simulink model "scheme_pos_control_yawcontrol"  (R2025a)
settings: Solver=ode3  StartTime=0.0  StopTime=40  FixedStep=dt  RelTol=1e-3
values from neighbouring files (symbols this model uses):
  dt = 0.0005    [Planning_Sim.m]
  goal_pos = waypoints(end, :)'    [Planning_Sim.m]
  initial_positions_rad = rawJointPositions(1, :)'    [manipulator_sim.m]
  manipulator_position_data = positions_final    [manipulator_sim.m]
  manipulator_time_vector = time_final    [manipulator_sim.m]
  map_scale = 0.5    [Planning_Sim.m]
  op_space_pose_trajectory = zeros(4, 4, num_points)    [Planning_Sim.m]
  waypoints = pathObj.States(:, 1:2)    [Planning_Sim.m]
  x0 = zeros(14, 1)    [Planning_Sim.m]
undefined symbols (not defined in the file or in its folder): control_params, p, X, Y, Z
libraries: sm_lib x179, nesl_utility x28, fl_lib x3
(part 1 of 5)
settings Model: SimulationMode=accelerator  Creator=robyr  LastModifiedBy=robyr
settings SolverCC: MinimalZcImpactIntegration=on
settings DebuggingCC: ReadBeforeWriteMsg=DisableAll  WriteAfterWriteMsg=DisableAll  WriteAfterReadMsg=DisableAll  MultiTaskDSMMsg=none
settings ModelReferenceCC: UpdateModelReferenceTargets=IfOutOfDate
settings SFSimCC: SFSimEcho=off
settings ExplorerConfigSet: InternalSimMechanicsExplorerSettings="<ExplorerConfiguration><canonicalview>default</canonicalview><TilePanel><TileInfo><Tiles Columns=\"1\" Count=\"1\" Height=\"983\" Rows=\"1\" Width=\"1140\"><Row Weight=\"1\"/><Column Weight=\"1\"/><Tile Height=\"1\" Width=\"1\" X=\"0\" Y=\"0\"/></Tiles></TileInfo><SceneInfo><SceneViewer><IsThisViewStd><IsStandardView>off</IsStandardView><StandardViewName>Front</StandardViewName></IsThisViewStd><BGColor><R>1</R><G>1</G><B>1</B><A>1</A></BGColor><Camera><DoPerspective>off</DoPerspective><Position><X>16.516580000000001</X><Y>-15.49729</Y><Z>6.32498</Z></Position><Center><X>0.84182000000000001</X><Y>-0.041480000000000003</Y><Z>0.82340999999999998</Z></Center><Up><X>0.26359755665786838</X><Y>0.54953240075907739</Y><Z>0.79279913511555156</Z></Up><XLim>1.6166905375218092</XLim><YLim>1.6166905375218092</YLim><ViewLimDist>0.01</ViewLimDist></Camera></SceneViewer></SceneInfo></TilePanel><MechEditorPanel><GfxPanelCameraMap/><Cameras/><VideoCreator><IncludeTiles>All</IncludeTiles><IncludeTime>on</IncludeTime><IncludeWorldFrame>off</IncludeWorldFrame><PlaybackSpeedRatio>1</PlaybackSpeedRatio><FrameRate>30</FrameRate><FrameSize>auto</FrameSize><VideoFormat>UncompressedAVI</VideoFormat></VideoCreator></MechEditorPanel><PlaybackSettings><PlaybackSpeedFactor>4</PlaybackSpeedFactor></PlaybackSettings></ExplorerConfiguration>"

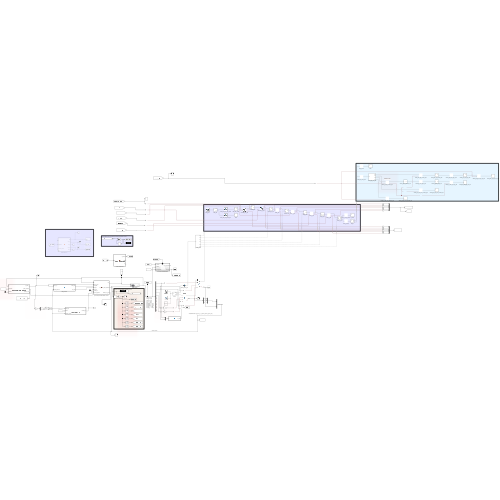
[thumbnail: Simulink's stored preview of the top-level diagram]
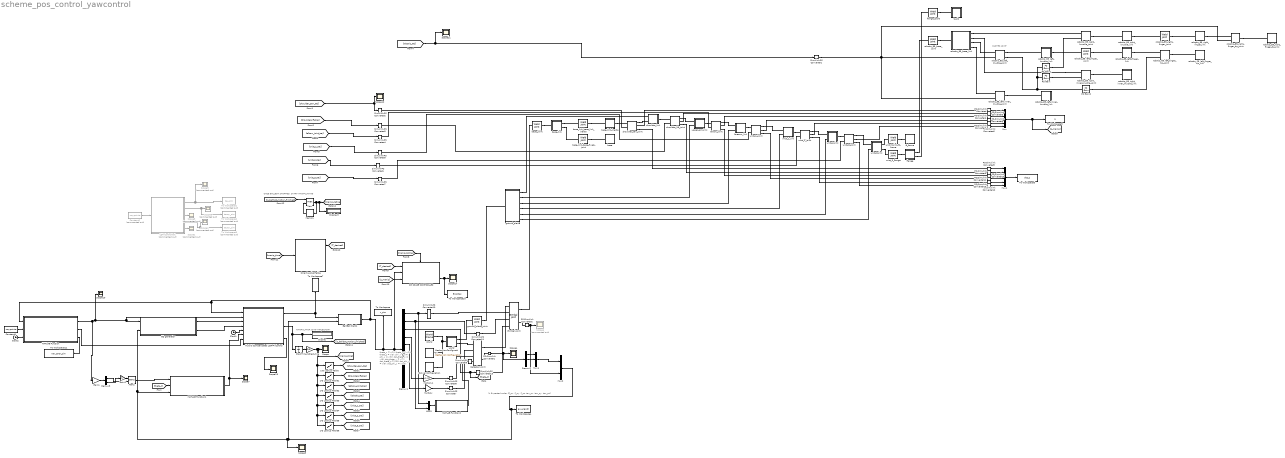
== system scheme_pos_control_yawcontrol ==
  note: MANIPULATOR JOINT TRAJECTORY
  note: % Expected order: [F_px, F_py, F_pz, tau_px, tau_py, tau_pz]
  note: theta_x = x(1);
      | theta_y = x(2);
      | theta_z = x(3);
      | phi_x = x(4);
      | phi_y = x(5);
      | dot_theta_x = x(6);
      | dot_theta_y = x(7);
      | dot_theta_z = x(8);
      | dot_phi_x = x(9);
      | dot_phi_y = x(10);
  note: MASTER JOINT
  note: ONCE BALLBOT STOPPED, START MANIPULATING
  1-D Lookup Table : Lookup_n-D  NumberOfTableDimensions=1  BreakpointsForDimension1=manipulator_time_vector  Table=manipulator_position_data(:,1)  InternalRulePriority=Speed  RndMeth=Simplest
  1-D Lookup Table1 : Lookup_n-D  NumberOfTableDimensions=1  BreakpointsForDimension1=manipulator_time_vector  Table=manipulator_position_data(:,2)  InternalRulePriority=Speed  RndMeth=Simplest
  1-D Lookup Table2 : Lookup_n-D  NumberOfTableDimensions=1  BreakpointsForDimension1=manipulator_time_vector  Table=manipulator_position_data(:,3)  InternalRulePriority=Speed  RndMeth=Simplest
  1-D Lookup Table3 : Lookup_n-D  NumberOfTableDimensions=1  BreakpointsForDimension1=manipulator_time_vector  Table=manipulator_position_data(:,4)  InternalRulePriority=Speed  RndMeth=Simplest
  1-D Lookup Table4 : Lookup_n-D  NumberOfTableDimensions=1  BreakpointsForDimension1=manipulator_time_vector  Table=manipulator_position_data(:,5)  InternalRulePriority=Speed  RndMeth=Simplest
  1-D Lookup Table5 : Lookup_n-D  NumberOfTableDimensions=1  BreakpointsForDimension1=manipulator_time_vector  Table=manipulator_position_data(:,6)  InternalRulePriority=Speed  RndMeth=Simplest
  1-D Lookup Table6 : Lookup_n-D  NumberOfTableDimensions=1  BreakpointsForDimension1=manipulator_time_vector  Table=manipulator_position_data(:,7)  InternalRulePriority=Speed  RndMeth=Simplest
  Atan2 : Trigonometry  Operator=atan2
  BallBot Plant1 : Subsystem
  Cartesian Joint : sm_lib/Joints/Cartesian Joint  JointMode=Normal  CompositeWrenchDir=FollowerOnBase  CompositeWrenchFrame=BaseFrame  SenseConstraintForce=off  SenseConstraintTorque=off  SenseTotalForce=on  SenseTotalTorque=off  PxPositionTargetSpecify=on  PxPositionTargetPriority=High  PxPositionTargetValue=0  PxPositionTargetValueUnits=m  PxVelocityTargetSpecify=on  PxVelocityTargetPriority=High  PxVelocityTargetValue=0  PxVelocityTargetValueUnits=m/s  PxEquilibriumPosition=0  PxEquilibriumPositionUnits=m  PxSpringStiffness=0  PxSpringStiffnessUnits=N/m  PxDampingCoefficient=0  PxDampingCoefficientUnits=N/(m/s)  PxLowerLimitSpecify=off  PxLowerLimitBound=-1  PxLowerLimitBoundUnits=m  PxLowerLimitStiffness=1e6  PxLowerLimitStiffnessUnits=N/m  PxLowerLimitDamping=1e3  PxLowerLimitDampingUnits=N/(m/s)  PxLowerLimitTransitionRegionWidth=1e-4  PxLowerLimitTransitionRegionWidthUnits=m  PxUpperLimitSpecify=off  PxUpperLimitBound=1  PxUpperLimitBoundUnits=m  PxUpperLimitStiffness=1e6  PxUpperLimitStiffnessUnits=N/m  PxUpperLimitDamping=1e3  PxUpperLimitDampingUnits=N/(m/s)  PxUpperLimitTransitionRegionWidth=1e-4  PxUpperLimitTransitionRegionWidthUnits=m  PxTorqueActuationMode=ComputedTorque  PxMotionActuationMode=InputMotion  PxSensePosition=off  PxSenseVelocity=off  PxSenseAcceleration=off  PxSenseTorqueForce=off  PxSenseLowerLimitTorqueForce=off  PxSenseUpperLimitTorqueForce=off  PyPositionTargetSpecify=on  PyPositionTargetPriority=High  PyPositionTargetValue=0  PyPositionTargetValueUnits=m  PyVelocityTargetSpecify=on  PyVelocityTargetPriority=High  PyVelocityTargetValue=0  PyVelocityTargetValueUnits=m/s  PyEquilibriumPosition=0  PyEquilibriumPositionUnits=m  PySpringStiffness=0  PySpringStiffnessUnits=N/m  PyDampingCoefficient=0  PyDampingCoefficientUnits=N/(m/s)  PyLowerLimitSpecify=off  PyLowerLimitBound=-1  PyLowerLimitBoundUnits=m  PyLowerLimitStiffness=1e6  PyLowerLimitStiffnessUnits=N/m  PyLowerLimitDamping=1e3  PyLowerLimitDampingUnits=N/(m/s)  PyLowerLimitTransitionRegionWidth=1e-4  PyLowerLimitTransitionRegionWidthUnits=m  PyUpperLimitSpecify=off  PyUpperLimitBound=1  PyUpperLimitBoundUnits=m  PyUpperLimitStiffness=1e6  PyUpperLimitStiffnessUnits=N/m  PyUpperLimitDamping=1e3  PyUpperLimitDampingUnits=N/(m/s)  PyUpperLimitTransitionRegionWidth=1e-4  PyUpperLimitTransitionRegionWidthUnits=m  PyTorqueActuationMode=ComputedTorque  PyMotionActuationMode=InputMotion  PySensePosition=off  PySenseVelocity=off  PySenseAcceleration=off  PySenseTorqueForce=off  PySenseLowerLimitTorqueForce=off  PySenseUpperLimitTorqueForce=off  PzPositionTargetSpecify=on  PzPositionTargetPriority=High  PzPositionTargetValue=0  PzPositionTargetValueUnits=m  PzVelocityTargetSpecify=on  PzVelocityTargetPriority=High  PzVelocityTargetValue=0  PzVelocityTargetValueUnits=m/s  PzEquilibriumPosition=0  PzEquilibriumPositionUnits=m  PzSpringStiffness=0  PzSpringStiffnessUnits=N/m  PzDampingCoefficient=0  PzDampingCoefficientUnits=N/(m/s)  PzLowerLimitSpecify=off  PzLowerLimitBound=-1  PzLowerLimitBoundUnits=m  PzLowerLimitStiffness=1e6  PzLowerLimitStiffnessUnits=N/m  PzLowerLimitDamping=1e3  PzLowerLimitDampingUnits=N/(m/s)  PzLowerLimitTransitionRegionWidth=1e-4  PzLowerLimitTransitionRegionWidthUnits=m  PzUpperLimitSpecify=off  PzUpperLimitBound=1  PzUpperLimitBoundUnits=m  PzUpperLimitStiffness=1e6  PzUpperLimitStiffnessUnits=N/m  PzUpperLimitDamping=1e3  PzUpperLimitDampingUnits=N/(m/s)  PzUpperLimitTransitionRegionWidth=1e-4  PzUpperLimitTransitionRegionWidthUnits=m  PzTorqueActuationMode=ComputedTorque  PzMotionActuationMode=InputMotion  PzSensePosition=off  PzSenseVelocity=off  PzSenseAcceleration=off  PzSenseTorqueForce=off  PzSenseLowerLimitTorqueForce=off  PzSenseUpperLimitTorqueForce=off
  Clock : Integrator
  Clock1 : Clock
  Clock2 : Clock
  Constant1 : Constant  Value=waypoints
  Constant6 : Constant  Commented=on  Value=waypoints
  Demux1 : Demux  Outputs=10
  Demux2 : Demux  Outputs=3
  Demux3 : Demux  Outputs=2
  Display : Display
  Display3 : Display
  EQ generator : MATLAB Function  TreatAsAtomicUnit=on
  Gain1 : Gain  Gain=p.r_S
  Gain2 : Gain
  Gimbal Joint : sm_lib/Joints/Gimbal Joint  JointMode=Normal  CompositeWrenchDir=FollowerOnBase  CompositeWrenchFrame=BaseFrame  SenseConstraintForce=off  SenseConstraintTorque=off  SenseTotalForce=off  SenseTotalTorque=on  RxPositionTargetSpecify=on  RxPositionTargetPriority=High  RxPositionTargetValue=0  RxPositionTargetValueUnits=deg  RxVelocityTargetSpecify=on  RxVelocityTargetPriority=High  RxVelocityTargetValue=0  RxVelocityTargetValueUnits=deg/s  RxEquilibriumPosition=0  RxEquilibriumPositionUnits=deg  RxSpringStiffness=0  RxSpringStiffnessUnits=N*m/deg  RxDampingCoefficient=0  RxDampingCoefficientUnits=N*m/(deg/s)  RxLowerLimitSpecify=off  RxLowerLimitBound=-90  RxLowerLimitBoundUnits=deg  RxLowerLimitStiffness=1e4  RxLowerLimitStiffnessUnits=N*m/deg  RxLowerLimitDamping=10  RxLowerLimitDampingUnits=N*m/(deg/s)  RxLowerLimitTransitionRegionWidth=0.1  RxLowerLimitTransitionRegionWidthUnits=deg  RxUpperLimitSpecify=off  RxUpperLimitBound=90  RxUpperLimitBoundUnits=deg  RxUpperLimitStiffness=1e4  RxUpperLimitStiffnessUnits=N*m/deg  RxUpperLimitDamping=10  RxUpperLimitDampingUnits=N*m/(deg/s)  RxUpperLimitTransitionRegionWidth=0.1  RxUpperLimitTransitionRegionWidthUnits=deg  RxTorqueActuationMode=ComputedTorque  RxMotionActuationMode=InputMotion  RxSensePosition=off  RxSenseVelocity=off  RxSenseAcceleration=off  RxSenseTorqueForce=off  RxSenseLowerLimitTorqueForce=off  RxSenseUpperLimitTorqueForce=off  RyPositionTargetSpecify=on  RyPositionTargetPriority=High  RyPositionTargetValue=0  RyPositionTargetValueUnits=deg  RyVelocityTargetSpecify=on  RyVelocityTargetPriority=High  RyVelocityTargetValue=0  RyVelocityTargetValueUnits=deg/s  RyEquilibriumPosition=0  RyEquilibriumPositionUnits=deg  RySpringStiffness=0  RySpringStiffnessUnits=N*m/deg  RyDampingCoefficient=0  RyDampingCoefficientUnits=N*m/(deg/s)  RyLowerLimitSpecify=off  RyLowerLimitBound=-90  RyLowerLimitBoundUnits=deg  RyLowerLimitStiffness=1e4  RyLowerLimitStiffnessUnits=N*m/deg  RyLowerLimitDamping=10  RyLowerLimitDampingUnits=N*m/(deg/s)  RyLowerLimitTransitionRegionWidth=0.1  RyLowerLimitTransitionRegionWidthUnits=deg  RyUpperLimitSpecify=off  RyUpperLimitBound=90  RyUpperLimitBoundUnits=deg  RyUpperLimitStiffness=1e4  RyUpperLimitStiffnessUnits=N*m/deg  RyUpperLimitDamping=10  RyUpperLimitDampingUnits=N*m/(deg/s)  RyUpperLimitTransitionRegionWidth=0.1  RyUpperLimitTransitionRegionWidthUnits=deg  RyTorqueActuationMode=ComputedTorque  RyMotionActuationMode=InputMotion  RySensePosition=off  RySenseVelocity=off  RySenseAcceleration=off  RySenseTorqueForce=off  RySenseLowerLimitTorqueForce=off  RySenseUpperLimitTorqueForce=off  RzPositionTargetSpecify=on  RzPositionTargetPriority=High  RzPositionTargetValue=0  RzPositionTargetValueUnits=deg  RzVelocityTargetSpecify=on  RzVelocityTargetPriority=High  RzVelocityTargetValue=0  RzVelocityTargetValueUnits=deg/s  RzEquilibriumPosition=0  RzEquilibriumPositionUnits=deg  RzSpringStiffness=0  RzSpringStiffnessUnits=N*m/deg  RzDampingCoefficient=0  RzDampingCoefficientUnits=N*m/(deg/s)  RzLowerLimitSpecify=off  RzLowerLimitBound=-90  RzLowerLimitBoundUnits=deg  RzLowerLimitStiffness=1e4  RzLowerLimitStiffnessUnits=N*m/deg  RzLowerLimitDamping=10  RzLowerLimitDampingUnits=N*m/(deg/s)  RzLowerLimitTransitionRegionWidth=0.1  RzLowerLimitTransitionRegionWidthUnits=deg  RzUpperLimitSpecify=off  RzUpperLimitBound=90  RzUpperLimitBoundUnits=deg  RzUpperLimitStiffness=1e4  RzUpperLimitStiffnessUnits=N*m/deg  RzUpperLimitDamping=10  RzUpperLimitDampingUnits=N*m/(deg/s)  RzUpperLimitTransitionRegionWidth=0.1  RzUpperLimitTransitionRegionWidthUnits=deg  RzTorqueActuationMode=ComputedTorque  RzMotionActuationMode=InputMotion  RzSensePosition=off  RzSenseVelocity=off  RzSenseAcceleration=off  RzSenseTorqueForce=off  RzSenseLowerLimitTorqueForce=off  RzSenseUpperLimitTorqueForce=off
  Hybrid Compensated LQR-PI Control : MATLAB Function  TreatAsAtomicUnit=on
  LQR Controller1 : MATLAB Function  Commented=on  TreatAsAtomicUnit=on
  MATLAB Function : MATLAB Function  TreatAsAtomicUnit=on
  MATLAB Function1 : MATLAB Function  TreatAsAtomicUnit=on
  MATLAB Function2 : MATLAB Function  TreatAsAtomicUnit=on
  Max : MinMax  Function=max  Inputs=2
  MechanismConfiguration : sm_lib/Utilities/Mechanism Configuration  UniformGravity=Constant  GravityVector=[0, 0, -9]  GravityVectorUnits=m/s^2  LinearizationDelta=0.001  JointModeTransitionNonlinearIterations=2
  Memory : Memory
  Multiply : Gain  Gain=p.r_S
  Multiply1 : Gain  Gain=-p.r_S
  Mux : Mux  Inputs=6
  Mux1 : Mux  Inputs=6
  Mux2 : Mux  Inputs=2
  Mux3 : Mux  Inputs=2
  Mux4 : Mux  Inputs=3
  OP SPACE CONTROLLER : Subsystem  TreatAsAtomicUnit=on
  PS Gain : fl_lib/Physical Signals/Functions/PS Gain  gain=-1
  PS Gain1 : fl_lib/Physical Signals/Functions/PS Gain  gain=-1
  PS Gain2 : fl_lib/Physical Signals/Functions/PS Gain  gain=-1
  PS-Simulink Converter{,1..13} (14 alike) : nesl_utility/PS-Simulink Converter  PhysicalDomain=network_engine_domain  SubClassName=ps_output  LeftPortType=input  RightPortType=output  PseudoPeriodic=off  Frequencies=[]  VectorFormat=inherit  Unit=inherit  AffineConversion=off
  Scope{,4..5,7,10..13,17} (9 alike) : Scope
      Scope settings: ActiveDisplayYMinimum=-1.1401390540569754  ActiveDisplayYMaximum=13.793855335305107  DataLoggingVariableName=ScopeData8
      Scope10 settings: ActiveDisplayYMinimum=-3.2555748380332981  ActiveDisplayYMaximum=3.1042480768285494  DataLoggingVariableName=ScopeData7
      Scope11 settings: ActiveDisplayYMinimum=-1  ActiveDisplayYMaximum=1  DataLoggingVariableName=ScopeData9
      Scope12 settings: ActiveDisplayYMinimum=-0.00099203829809874034  ActiveDisplayYMaximum=0.00011022647756651233  DataLoggingVariableName=ScopeData10
      Scope13 settings: ActiveDisplayYMinimum=-0.75168785516115677  ActiveDisplayYMaximum=6.7790572620323619  DataLoggingVariableName=ScopeData12
      Scope17 settings: ActiveDisplayYMinimum=-0.16810485018053126  ActiveDisplayYMaximum=0.21531354151049178  DataLoggingVariableName=ScopeData14
      Scope4 settings: ActiveDisplayYMinimum=-268.72143096974315  ActiveDisplayYMaximum=329.02280832847254  DataLoggingVariableName=ScopeData19
      Scope5 settings: ActiveDisplayYMinimum=-51.484934044784  ActiveDisplayYMaximum=102.53132354146534  DataLoggingVariableName=ScopeData4
      Scope7 settings: ActiveDisplayYMinimum=-2.2991535470315876  ActiveDisplayYMaximum=20.692381923284291  DataLoggingVariableName=ScopeData5
  Scope{1..3,6,8..9} (6 alike) : Scope  Commented=on
      Scope1 settings: ActiveDisplayYMinimum=-1.125  ActiveDisplayYMaximum=0.12499999999999997
      Scope2 settings: ActiveDisplayYMinimum=-1  ActiveDisplayYMaximum=1
      Scope3 settings: ActiveDisplayYMinimum=-0.1364286166044579  ActiveDisplayYMaximum=1.2278575494401214  DataLoggingVariableName=ScopeData3
      Scope6 settings: ActiveDisplayYMinimum=-20.564846798657925  ActiveDisplayYMaximum=40.294538035365044  DataLoggingVariableName=ScopeData21
      Scope8 settings: ActiveDisplayYMinimum=-1  ActiveDisplayYMaximum=1  DataLoggingVariableName=ScopeData2
      Scope9 settings: ActiveDisplayYMinimum=-1.1364286166044579  ActiveDisplayYMaximum=0.22785754944012135  DataLoggingVariableName=ScopeData6
  Simulink-PS Converter{,1..9,11,13} (12 alike) : nesl_utility/Simulink-PS Converter  PhysicalDomain=network_engine_domain  SubClassName=ps_input  LeftPortType=input  RightPortType=output  PseudoPeriodic=off  Frequencies=[]  NoiseDistribution=none  NoiseParameters=[]  Unit=1  AffineConversion=off  FilteringAndDerivatives=filter  SimscapeFilterOrder=2  InputFilterTimeConstant=0.001  UdotUserProvided=0
  Simulink-PS Converter10 : nesl_utility/Simulink-PS Converter  PhysicalDomain=network_engine_domain  SubClassName=ps_input  LeftPortType=input  RightPortType=output  PseudoPeriodic=off  Frequencies=[]  NoiseDistribution=none  NoiseParameters=[]  Unit=1  AffineConversion=off  FilteringAndDerivatives=filter  SimscapeFilterOrder=2  InputFilterTimeConstant=0.001  UdotUserProvided=2
  Smart LookUpTable : MATLAB Function  TreatAsAtomicUnit=on
  Solver Configuration : nesl_utility/Solver Configuration  PhysicalDomain=network_engine_domain  SubClassName=solver  LeftPortType=input  RightPortType=generic  Tones=[]  Harmonics=[]  SimulateNoise=off  Profile=off  UseLocalSampling=off  EnableSwitchedLinearOptims=on  FrequencyDomain=off  UseCCode=off  RelTol=0.001  AbsTol=0.001  MinStep=1e-09  ToWorkspace=off  RevertToSquareIcSolve=off  NumHomotopyIterations=100  PhasorMode=off  PhasorModeNumHarmonics=1  ConsistencySolver=NEWTON_XTOL_AFTER_FTOL  IndexReductionMethod=DerivativeReplacement  DoDC=off  ResidualTolerance=1e-09  ConsistencyTolSource=GLOBAL  ConsistencyAbsTol=0.001  ConsistencyRelTol=0.001  ConsistencyTolFactor=0.001  UseLocalSolver=off  LocalSolverChoice=NE_BACKWARD_EULER_ADVANCER  ResolveIndetEquations=on  FunctionEvalNumThread=1  LocalSolverSampleTime=0.001  DoFixedCost=off  MaxNonlinIter=3  MaxModeIter=2  ComputeImpulses=off  ImpulseIterations=2  LinearAlgebra=auto  LinearAlgebraNumThread=0  EquationFormulation=NE_TIME_EF  DelaysMemoryBudget=1024  AutomaticFiltering=on  FilteringTimeConstant=0.01  PartitionStorageMethod=AS_NEEDED  PartitionMemoryBudget=1024  PartitionMethod=ROBUST  MultibodyUseLocalSolver=off  MultibodyLocalSolverChoice=ODE1  MultibodyLocalSolverSampleTime=0.001
  Time Scheduling : Gain  Gain=1/5
  To Workspace : ToWorkspace  VariableName=x_sim  SaveFormat=Timeseries  SampleTime=-1
  To Workspace1 : ToWorkspace  Commented=on  VariableName=tau_sim  SaveFormat=Timeseries  SampleTime=-1
  To Workspace10 : ToWorkspace  VariableName=ErrorPos  SaveFormat=Timeseries  SampleTime=-1
  To Workspace11 : ToWorkspace  VariableName=nav_error_sim  SaveFormat=Timeseries  SampleTime=-1
  To Workspace2 : ToWorkspace  Commented=on  VariableName=tauey_sim  SaveFormat=Timeseries  SampleTime=-1
  To Workspace3 : ToWorkspace  Commented=on  VariableName=tauex_sim  SaveFormat=Timeseries  SampleTime=-1
  To Workspace4 : ToWorkspace  VariableName=ex_wrench  SaveFormat=Timeseries  SampleTime=-1
  To Workspace5 : ToWorkspace  VariableName=q  SaveFormat=Timeseries  SampleTime=-1
  To Workspace6 : ToWorkspace  VariableName=dot_q  SaveFormat=Timeseries  SampleTime=-1
  To Workspace7 : ToWorkspace  VariableName=tau_sim  SaveFormat=Timeseries  SampleTime=-1
  World : sm_lib/Frames and Transforms/World Frame
  base : Subsystem
  base_joint : sm_lib/Joints/Weld Joint  JointMode=Normal  CompositeWrenchDir=FollowerOnBase  CompositeWrenchFrame=BaseFrame  SenseConstraintForce=off  SenseConstraintTorque=off  SenseTotalForce=off  SenseTotalTorque=off
  base_link : Subsystem
  base_link_base_fixed_joint : sm_lib/Joints/Weld Joint  JointMode=Normal  CompositeWrenchDir=FollowerOnBase  CompositeWrenchFrame=BaseFrame  SenseConstraintForce=off  SenseConstraintTorque=off  SenseTotalForce=off  SenseTotalTorque=off
  base_link_base_link_inertia : sm_lib/Joints/Weld Joint  JointMode=Normal  CompositeWrenchDir=FollowerOnBase  CompositeWrenchFrame=BaseFrame  SenseConstraintForce=off  SenseConstraintTorque=off  SenseTotalForce=off  SenseTotalTorque=off
  base_link_inertia : Subsystem
  elbow_joint : sm_lib/Joints/Revolute Joint  JointMode=Normal  CompositeWrenchDir=FollowerOnBase  CompositeWrenchFrame=BaseFrame  SenseConstraintForce=off  SenseConstraintTorque=off  SenseTotalForce=off  SenseTotalTorque=off  PositionTargetSpecify=on  PositionTargetPriority=High  PositionTargetValue=2.3560  PositionTargetValueUnits=rad  VelocityTargetSpecify=off  VelocityTargetPriority=High  VelocityTargetValue=0  VelocityTargetValueUnits=deg/s  EquilibriumPosition=0  EquilibriumPositionUnits=deg  SpringStiffness=0  SpringStiffnessUnits=N*m/deg  DampingCoefficient=0  DampingCoefficientUnits=kg*m^2/(rad*s)  LowerLimitSpecify=off  LowerLimitBound=-3.141592653589793  LowerLimitBoundUnits=rad  LowerLimitStiffness=1e4  LowerLimitStiffnessUnits=N*m/deg  LowerLimitDamping=10  LowerLimitDampingUnits=N*m/(deg/s)  LowerLimitTransitionRegionWidth=0.1  LowerLimitTransitionRegionWidthUnits=deg  UpperLimitSpecify=off  UpperLimitBound=3.141592653589793  UpperLimitBoundUnits=rad  UpperLimitStiffness=1e4  UpperLimitStiffnessUnits=N*m/deg  UpperLimitDamping=10  UpperLimitDampingUnits=N*m/(deg/s)  UpperLimitTransitionRegionWidth=0.1  UpperLimitTransitionRegionWidthUnits=deg  TorqueActuationMode=ComputedTorque  MotionActuationMode=InputMotion  SensePosition=on  SenseVelocity=on  SenseAcceleration=off  SenseTorqueForce=off  SenseLowerLimitTorqueForce=off  SenseUpperLimitTorqueForce=off
  flange : Subsystem
  flange_tool0 : sm_lib/Joints/Weld Joint  JointMode=Normal  CompositeWrenchDir=FollowerOnBase  CompositeWrenchFrame=BaseFrame  SenseConstraintForce=off  SenseConstraintTorque=off  SenseTotalForce=off  SenseTotalTorque=off
  forearm_link : Subsystem
  ft_frame : Subsystem
  ground_plane : Subsystem
  ground_plane_joint : sm_lib/Joints/Weld Joint  JointMode=Normal  CompositeWrenchDir=FollowerOnBase  CompositeWrenchFrame=BaseFrame  SenseConstraintForce=off  SenseConstraintTorque=off  SenseTotalForce=off  SenseTotalTorque=off
  robotiq_85_base_joint : sm_lib/Joints/Weld Joint  JointMode=Normal  CompositeWrenchDir=FollowerOnBase  CompositeWrenchFrame=BaseFrame  SenseConstraintForce=off  SenseConstraintTorque=off  SenseTotalForce=off  SenseTotalTorque=off
  robotiq_85_base_link : Subsystem
  robotiq_85_left_finger_joint : sm_lib/Joints/Weld Joint  JointMode=Normal  CompositeWrenchDir=FollowerOnBase  CompositeWrenchFrame=BaseFrame  SenseConstraintForce=off  SenseConstraintTorque=off  SenseTotalForce=off  SenseTotalTorque=off
  robotiq_85_left_finger_link : Subsystem
  robotiq_85_left_finger_tip_joint : sm_lib/Joints/Revolute Joint  JointMode=Normal  CompositeWrenchDir=FollowerOnBase  CompositeWrenchFrame=BaseFrame  SenseConstraintForce=off  SenseConstraintTorque=off  SenseTotalForce=off  SenseTotalTorque=off  PositionTargetSpecify=on  PositionTargetPriority=High  PositionTargetValue=0  PositionTargetValueUnits=rad  VelocityTargetSpecify=off  VelocityTargetPriority=High  VelocityTargetValue=0  VelocityTargetValueUnits=deg/s  EquilibriumPosition=0  EquilibriumPositionUnits=deg  SpringStiffness=0  SpringStiffnessUnits=N*m/deg  DampingCoefficient=0  DampingCoefficientUnits=kg*m^2/(rad*s)  LowerLimitSpecify=off  LowerLimitBound=-90  LowerLimitBoundUnits=deg  LowerLimitStiffness=1e4  LowerLimitStiffnessUnits=N*m/deg  LowerLimitDamping=10  LowerLimitDampingUnits=N*m/(deg/s)  LowerLimitTransitionRegionWidth=0.1  LowerLimitTransitionRegionWidthUnits=deg  UpperLimitSpecify=off  UpperLimitBound=90  UpperLimitBoundUnits=deg  UpperLimitStiffness=1e4  UpperLimitStiffnessUnits=N*m/deg  UpperLimitDamping=10  UpperLimitDampingUnits=N*m/(deg/s)  UpperLimitTransitionRegionWidth=0.1  UpperLimitTransitionRegionWidthUnits=deg  TorqueActuationMode=ComputedTorque  MotionActuationMode=InputMotion  SensePosition=off  SenseVelocity=off  SenseAcceleration=off  SenseTorqueForce=off  SenseLowerLimitTorqueForce=off  SenseUpperLimitTorqueForce=off
  robotiq_85_left_finger_tip_link : Subsystem
  robotiq_85_left_inner_knuckle_joint : sm_lib/Joints/Revolute Joint  JointMode=Normal  CompositeWrenchDir=FollowerOnBase  CompositeWrenchFrame=BaseFrame  SenseConstraintForce=off  SenseConstraintTorque=off  SenseTotalForce=off  SenseTotalTorque=off  PositionTargetSpecify=off  PositionTargetPriority=High  PositionTargetValue=0  PositionTargetValueUnits=rad  VelocityTargetSpecify=off  VelocityTargetPriority=High  VelocityTargetValue=0  VelocityTargetValueUnits=deg/s  EquilibriumPosition=0  EquilibriumPositionUnits=deg  SpringStiffness=0  SpringStiffnessUnits=N*m/deg  DampingCoefficient=0  DampingCoefficientUnits=kg*m^2/(rad*s)  LowerLimitSpecify=off  LowerLimitBound=-90  LowerLimitBoundUnits=deg  LowerLimitStiffness=1e4  LowerLimitStiffnessUnits=N*m/deg  LowerLimitDamping=10  LowerLimitDampingUnits=N*m/(deg/s)  LowerLimitTransitionRegionWidth=0.1  LowerLimitTransitionRegionWidthUnits=deg  UpperLimitSpecify=off  UpperLimitBound=90  UpperLimitBoundUnits=deg  UpperLimitStiffness=1e4  UpperLimitStiffnessUnits=N*m/deg  UpperLimitDamping=10  UpperLimitDampingUnits=N*m/(deg/s)  UpperLimitTransitionRegionWidth=0.1  UpperLimitTransitionRegionWidthUnits=deg  TorqueActuationMode=ComputedTorque  MotionActuationMode=InputMotion  SensePosition=off  SenseVelocity=off  SenseAcceleration=off  SenseTorqueForce=off  SenseLowerLimitTorqueForce=off  SenseUpperLimitTorqueForce=off
  robotiq_85_left_inner_knuckle_link : Subsystem
  robotiq_85_left_knuckle_joint : sm_lib/Joints/Revolute Joint  JointMode=Normal  CompositeWrenchDir=FollowerOnBase  CompositeWrenchFrame=BaseFrame  SenseConstraintForce=off  SenseConstraintTorque=off  SenseTotalForce=off  SenseTotalTorque=off  PositionTargetSpecify=on  PositionTargetPriority=High  PositionTargetValue=initial_positions_rad(4)  PositionTargetValueUnits=rad  VelocityTargetSpecify=off  VelocityTargetPriority=High  VelocityTargetValue=0  VelocityTargetValueUnits=deg/s  EquilibriumPosition=0  EquilibriumPositionUnits=deg  SpringStiffness=0  SpringStiffnessUnits=N*m/deg  DampingCoefficient=0  DampingCoefficientUnits=kg*m^2/(rad*s)  LowerLimitSpecify=on  LowerLimitBound=0  LowerLimitBoundUnits=rad  LowerLimitStiffness=1e4  LowerLimitStiffnessUnits=N*m/deg  LowerLimitDamping=10  LowerLimitDampingUnits=N*m/(deg/s)  LowerLimitTransitionRegionWidth=0.1  LowerLimitTransitionRegionWidthUnits=deg  UpperLimitSpecify=on  UpperLimitBound=0.8  UpperLimitBoundUnits=rad  UpperLimitStiffness=1e4  UpperLimitStiffnessUnits=N*m/deg  UpperLimitDamping=10  UpperLimitDampingUnits=N*m/(deg/s)  UpperLimitTransitionRegionWidth=0.1  UpperLimitTransitionRegionWidthUnits=deg  TorqueActuationMode=ComputedTorque  MotionActuationMode=InputMotion  SensePosition=on  SenseVelocity=off  SenseAcceleration=off  SenseTorqueForce=off  SenseLowerLimitTorqueForce=off  SenseUpperLimitTorqueForce=off
  robotiq_85_left_knuckle_link : Subsystem
  robotiq_85_right_finger_joint : sm_lib/Joints/Weld Joint  JointMode=Normal  CompositeWrenchDir=FollowerOnBase  CompositeWrenchFrame=BaseFrame  SenseConstraintForce=off  SenseConstraintTorque=off  SenseTotalForce=off  SenseTotalTorque=off
  robotiq_85_right_finger_link : Subsystem
  robotiq_85_right_finger_tip_joint : sm_lib/Joints/Revolute Joint  JointMode=Normal  CompositeWrenchDir=FollowerOnBase  CompositeWrenchFrame=BaseFrame  SenseConstraintForce=off  SenseConstraintTorque=off  SenseTotalForce=off  SenseTotalTorque=off  PositionTargetSpecify=on  PositionTargetPriority=High  PositionTargetValue=0  PositionTargetValueUnits=rad  VelocityTargetSpecify=off  VelocityTargetPriority=High  VelocityTargetValue=0  VelocityTargetValueUnits=deg/s  EquilibriumPosition=0  EquilibriumPositionUnits=deg  SpringStiffness=0  SpringStiffnessUnits=N*m/deg  DampingCoefficient=0  DampingCoefficientUnits=kg*m^2/(rad*s)  LowerLimitSpecify=off  LowerLimitBound=-90  LowerLimitBoundUnits=deg  LowerLimitStiffness=1e4  LowerLimitStiffnessUnits=N*m/deg  LowerLimitDamping=10  LowerLimitDampingUnits=N*m/(deg/s)  LowerLimitTransitionRegionWidth=0.1  LowerLimitTransitionRegionWidthUnits=deg  UpperLimitSpecify=off  UpperLimitBound=90  UpperLimitBoundUnits=deg  UpperLimitStiffness=1e4  UpperLimitStiffnessUnits=N*m/deg  UpperLimitDamping=10  UpperLimitDampingUnits=N*m/(deg/s)  UpperLimitTransitionRegionWidth=0.1  UpperLimitTransitionRegionWidthUnits=deg  TorqueActuationMode=ComputedTorque  MotionActuationMode=InputMotion  SensePosition=off  SenseVelocity=off  SenseAcceleration=off  SenseTorqueForce=off  SenseLowerLimitTorqueForce=off  SenseUpperLimitTorqueForce=off
  robotiq_85_right_finger_tip_link : Subsystem
  robotiq_85_right_inner_knuckle_joint : sm_lib/Joints/Revolute Joint  JointMode=Normal  CompositeWrenchDir=FollowerOnBase  CompositeWrenchFrame=BaseFrame  SenseConstraintForce=off  SenseConstraintTorque=off  SenseTotalForce=off  SenseTotalTorque=off  PositionTargetSpecify=off  PositionTargetPriority=High  PositionTargetValue=0  PositionTargetValueUnits=rad  VelocityTargetSpecify=off  VelocityTargetPriority=High  VelocityTargetValue=0  VelocityTargetValueUnits=deg/s  EquilibriumPosition=0  EquilibriumPositionUnits=deg  SpringStiffness=0  SpringStiffnessUnits=N*m/deg  DampingCoefficient=0  DampingCoefficientUnits=kg*m^2/(rad*s)  LowerLimitSpecify=off  LowerLimitBound=-90  LowerLimitBoundUnits=deg  LowerLimitStiffness=1e4  LowerLimitStiffnessUnits=N*m/deg  LowerLimitDamping=10  LowerLimitDampingUnits=N*m/(deg/s)  LowerLimitTransitionRegionWidth=0.1  LowerLimitTransitionRegionWidthUnits=deg  UpperLimitSpecify=off  UpperLimitBound=90  UpperLimitBoundUnits=deg  UpperLimitStiffness=1e4  UpperLimitStiffnessUnits=N*m/deg  UpperLimitDamping=10  UpperLimitDampingUnits=N*m/(deg/s)  UpperLimitTransitionRegionWidth=0.1  UpperLimitTransitionRegionWidthUnits=deg  TorqueActuationMode=ComputedTorque  MotionActuationMode=InputMotion  SensePosition=off  SenseVelocity=off  SenseAcceleration=off  SenseTorqueForce=off  SenseLowerLimitTorqueForce=off  SenseUpperLimitTorqueForce=off
  robotiq_85_right_inner_knuckle_link : Subsystem
  robotiq_85_right_knuckle_joint : sm_lib/Joints/Revolute Joint  JointMode=Normal  CompositeWrenchDir=FollowerOnBase  CompositeWrenchFrame=BaseFrame  SenseConstraintForce=off  SenseConstraintTorque=off  SenseTotalForce=off  SenseTotalTorque=off  PositionTargetSpecify=off  PositionTargetPriority=High  PositionTargetValue=0  PositionTargetValueUnits=rad  VelocityTargetSpecify=off  VelocityTargetPriority=High  VelocityTargetValue=0  VelocityTargetValueUnits=deg/s  EquilibriumPosition=0  EquilibriumPositionUnits=deg  SpringStiffness=0  SpringStiffnessUnits=N*m/deg  DampingCoefficient=0  DampingCoefficientUnits=kg*m^2/(rad*s)  LowerLimitSpecify=on  LowerLimitBound=-0.8  LowerLimitBoundUnits=rad  LowerLimitStiffness=1e4  LowerLimitStiffnessUnits=N*m/deg  LowerLimitDamping=10  LowerLimitDampingUnits=N*m/(deg/s)  LowerLimitTransitionRegionWidth=0.1  LowerLimitTransitionRegionWidthUnits=deg  UpperLimitSpecify=on  UpperLimitBound=0  UpperLimitBoundUnits=rad  UpperLimitStiffness=1e4  UpperLimitStiffnessUnits=N*m/deg  UpperLimitDamping=10  UpperLimitDampingUnits=N*m/(deg/s)  UpperLimitTransitionRegionWidth=0.1  UpperLimitTransitionRegionWidthUnits=deg  TorqueActuationMode=ComputedTorque  MotionActuationMode=InputMotion  SensePosition=off  SenseVelocity=off  SenseAcceleration=off  SenseTorqueForce=off  SenseLowerLimitTorqueForce=off  SenseUpperLimitTorqueForce=off
  robotiq_85_right_knuckle_link : Subsystem
  shoulder_lift_joint : sm_lib/Joints/Revolute Joint  JointMode=Normal  CompositeWrenchDir=FollowerOnBase  CompositeWrenchFrame=BaseFrame  SenseConstraintForce=off  SenseConstraintTorque=off  SenseTotalForce=off  SenseTotalTorque=off  PositionTargetSpecify=on  PositionTargetPriority=High  PositionTargetValue=-2.3560  PositionTargetValueUnits=rad  VelocityTargetSpecify=off  VelocityTargetPriority=High  VelocityTargetValue=0  VelocityTargetValueUnits=deg/s  EquilibriumPosition=0  EquilibriumPositionUnits=deg  SpringStiffness=0  SpringStiffnessUnits=N*m/deg  DampingCoefficient=0  DampingCoefficientUnits=kg*m^2/(rad*s)  LowerLimitSpecify=on  LowerLimitBound=-6.283185307179586  LowerLimitBoundUnits=rad  LowerLimitStiffness=1e4  LowerLimitStiffnessUnits=N*m/deg  LowerLimitDamping=10  LowerLimitDampingUnits=N*m/(deg/s)  LowerLimitTransitionRegionWidth=0.1  LowerLimitTransitionRegionWidthUnits=deg  UpperLimitSpecify=on  UpperLimitBound=6.283185307179586  UpperLimitBoundUnits=rad  UpperLimitStiffness=1e4  UpperLimitStiffnessUnits=N*m/deg  UpperLimitDamping=10  UpperLimitDampingUnits=N*m/(deg/s)  UpperLimitTransitionRegionWidth=0.1  UpperLimitTransitionRegionWidthUnits=deg  TorqueActuationMode=ComputedTorque  MotionActuationMode=InputMotion  SensePosition=on  SenseVelocity=on  SenseAcceleration=off  SenseTorqueForce=off  SenseLowerLimitTorqueForce=off  SenseUpperLimitTorqueForce=off
  shoulder_link : Subsystem
  shoulder_pan_joint : sm_lib/Joints/Revolute Joint  JointMode=Normal  CompositeWrenchDir=FollowerOnBase  CompositeWrenchFrame=BaseFrame  SenseConstraintForce=off  SenseConstraintTorque=off  SenseTotalForce=off  SenseTotalTorque=off  PositionTargetSpecify=on  PositionTargetPriority=High  PositionTargetValue=0  PositionTargetValueUnits=rad  VelocityTargetSpecify=off  VelocityTargetPriority=High  VelocityTargetValue=0  VelocityTargetValueUnits=deg/s  EquilibriumPosition=0  EquilibriumPositionUnits=deg  SpringStiffness=0  SpringStiffnessUnits=N*m/deg  DampingCoefficient=0  DampingCoefficientUnits=kg*m^2/(rad*s)  LowerLimitSpecify=on  LowerLimitBound=-6.283185307179586  LowerLimitBoundUnits=rad  LowerLimitStiffness=1e4  LowerLimitStiffnessUnits=N*m/deg  LowerLimitDamping=10  LowerLimitDampingUnits=N*m/(deg/s)  LowerLimitTransitionRegionWidth=0.1  LowerLimitTransitionRegionWidthUnits=deg  UpperLimitSpecify=on  UpperLimitBound=6.283185307179586  UpperLimitBoundUnits=rad  UpperLimitStiffness=1e4  UpperLimitStiffnessUnits=N*m/deg  UpperLimitDamping=10  UpperLimitDampingUnits=N*m/(deg/s)  UpperLimitTransitionRegionWidth=0.1  UpperLimitTransitionRegionWidthUnits=deg  TorqueActuationMode=ComputedTorque  MotionActuationMode=InputMotion  SensePosition=on  SenseVelocity=on  SenseAcceleration=off  SenseTorqueForce=off  SenseLowerLimitTorqueForce=off  SenseUpperLimitTorqueForce=off
  tool0 : Subsystem
  upper_arm_link : Subsystem
  world : Subsystem
  wrist_1_joint : sm_lib/Joints/Revolute Joint  JointMode=Normal  CompositeWrenchDir=FollowerOnBase  CompositeWrenchFrame=BaseFrame  SenseConstraintForce=off  SenseConstraintTorque=off  SenseTotalForce=off  SenseTotalTorque=off  PositionTargetSpecify=on  PositionTargetPriority=High  PositionTargetValue=-1.57  PositionTargetValueUnits=rad  VelocityTargetSpecify=off  VelocityTargetPriority=High  VelocityTargetValue=0  VelocityTargetValueUnits=deg/s  EquilibriumPosition=0  EquilibriumPositionUnits=deg  SpringStiffness=0  SpringStiffnessUnits=N*m/deg  DampingCoefficient=0  DampingCoefficientUnits=kg*m^2/(rad*s)  LowerLimitSpecify=on  LowerLimitBound=-6.283185307179586  LowerLimitBoundUnits=rad  LowerLimitStiffness=1e4  LowerLimitStiffnessUnits=N*m/deg  LowerLimitDamping=10  LowerLimitDampingUnits=N*m/(deg/s)  LowerLimitTransitionRegionWidth=0.1  LowerLimitTransitionRegionWidthUnits=deg  UpperLimitSpecify=on  UpperLimitBound=6.283185307179586  UpperLimitBoundUnits=rad  UpperLimitStiffness=1e4  UpperLimitStiffnessUnits=N*m/deg  UpperLimitDamping=10  UpperLimitDampingUnits=N*m/(deg/s)  UpperLimitTransitionRegionWidth=0.1  UpperLimitTransitionRegionWidthUnits=deg  TorqueActuationMode=ComputedTorque  MotionActuationMode=InputMotion  SensePosition=on  SenseVelocity=on  SenseAcceleration=off  SenseTorqueForce=off  SenseLowerLimitTorqueForce=off  SenseUpperLimitTorqueForce=off
  wrist_1_link : Subsystem
  wrist_2_joint : sm_lib/Joints/Revolute Joint  JointMode=Normal  CompositeWrenchDir=FollowerOnBase  CompositeWrenchFrame=BaseFrame  SenseConstraintForce=off  SenseConstraintTorque=off  SenseTotalForce=off  SenseTotalTorque=off  PositionTargetSpecify=on  PositionTargetPriority=High  PositionTargetValue=-1.57  PositionTargetValueUnits=rad  VelocityTargetSpecify=off  VelocityTargetPriority=High  VelocityTargetValue=0  VelocityTargetValueUnits=deg/s  EquilibriumPosition=0  EquilibriumPositionUnits=deg  SpringStiffness=0  SpringStiffnessUnits=N*m/deg  DampingCoefficient=0  DampingCoefficientUnits=kg*m^2/(rad*s)  LowerLimitSpecify=on  LowerLimitBound=-6.283185307179586  LowerLimitBoundUnits=rad  LowerLimitStiffness=1e4  LowerLimitStiffnessUnits=N*m/deg  LowerLimitDamping=10  LowerLimitDampingUnits=N*m/(deg/s)  LowerLimitTransitionRegionWidth=0.1  LowerLimitTransitionRegionWidthUnits=deg  UpperLimitSpecify=on  UpperLimitBound=6.283185307179586  UpperLimitBoundUnits=rad  UpperLimitStiffness=1e4  UpperLimitStiffnessUnits=N*m/deg  UpperLimitDamping=10  UpperLimitDampingUnits=N*m/(deg/s)  UpperLimitTransitionRegionWidth=0.1  UpperLimitTransitionRegionWidthUnits=deg  TorqueActuationMode=ComputedTorque  MotionActuationMode=InputMotion  SensePosition=on  SenseVelocity=on  SenseAcceleration=off  SenseTorqueForce=off  SenseLowerLimitTorqueForce=off  SenseUpperLimitTorqueForce=off
  wrist_2_link : Subsystem
  wrist_3_flange : sm_lib/Joints/Weld Joint  JointMode=Normal  CompositeWrenchDir=FollowerOnBase  CompositeWrenchFrame=BaseFrame  SenseConstraintForce=off  SenseConstraintTorque=off  SenseTotalForce=off  SenseTotalTorque=off
  wrist_3_joint : sm_lib/Joints/Revolute Joint  JointMode=Normal  CompositeWrenchDir=FollowerOnBase  CompositeWrenchFrame=BaseFrame  SenseConstraintForce=off  SenseConstraintTorque=off  SenseTotalForce=off  SenseTotalTorque=off  PositionTargetSpecify=on  PositionTargetPriority=High  PositionTargetValue=0  PositionTargetValueUnits=rad  VelocityTargetSpecify=off  VelocityTargetPriority=High  VelocityTargetValue=0  VelocityTargetValueUnits=deg/s  EquilibriumPosition=0  EquilibriumPositionUnits=deg  SpringStiffness=0  SpringStiffnessUnits=N*m/deg  DampingCoefficient=0  DampingCoefficientUnits=kg*m^2/(rad*s)  LowerLimitSpecify=on  LowerLimitBound=-6.283185307179586  LowerLimitBoundUnits=rad  LowerLimitStiffness=1e4  LowerLimitStiffnessUnits=N*m/deg  LowerLimitDamping=10  LowerLimitDampingUnits=N*m/(deg/s)  LowerLimitTransitionRegionWidth=0.1  LowerLimitTransitionRegionWidthUnits=deg  UpperLimitSpecify=on  UpperLimitBound=6.283185307179586  UpperLimitBoundUnits=rad  UpperLimitStiffness=1e4  UpperLimitStiffnessUnits=N*m/deg  UpperLimitDamping=10  UpperLimitDampingUnits=N*m/(deg/s)  UpperLimitTransitionRegionWidth=0.1  UpperLimitTransitionRegionWidthUnits=deg  TorqueActuationMode=ComputedTorque  MotionActuationMode=InputMotion  SensePosition=on  SenseVelocity=on  SenseAcceleration=off  SenseTorqueForce=off  SenseLowerLimitTorqueForce=off  SenseUpperLimitTorqueForce=off
  wrist_3_link : Subsystem
  wrist_3_link_ft_frame : sm_lib/Joints/Weld Joint  JointMode=Normal  CompositeWrenchDir=FollowerOnBase  CompositeWrenchFrame=BaseFrame  SenseConstraintForce=off  SenseConstraintTorque=off  SenseTotalForce=off  SenseTotalTorque=off
  wires:
  LQR Controller1/4(tau_ex) -> Scope2/1, To Workspace3/1
  LQR Controller1/2(tau_ey) -> Scope8/1, To Workspace2/1
  Demux1/3 -> [theta_z], Simulink-PS Converter13/1
  Demux1/4 -> Multiply1/1
  Demux1/5 -> Multiply/1
  Multiply1/1 -> Simulink-PS Converter8/1
  Multiply/1 -> Simulink-PS Converter/1
  PS-Simulink Converter2/1 -> Mux2/2, Scope6/1
  PS-Simulink Converter/1 -> Mux/1
  PS-Simulink Converter3/1 -> Mux/2
  PS-Simulink Converter4/1 -> Mux/3
  PS-Simulink Converter5/1 -> Mux/4
  PS-Simulink Converter6/1 -> Mux/5
  PS-Simulink Converter7/1 -> Mux/6
  Mux/1 -> [q_manip], To Workspace5/1
  Mux1/1 -> To Workspace6/1
  PS-Simulink Converter13/1 -> Mux1/6
  PS-Simulink Converter12/1 -> Mux1/5
  PS-Simulink Converter11/1 -> Mux1/4
  PS-Simulink Converter10/1 -> Mux1/3
  PS-Simulink Converter9/1 -> Mux1/2
  PS-Simulink Converter8/1 -> Mux1/1
  [robotiq_traj] -> Scope11/1, Simulink-PS Converter1/1
  Mux2/1 -> To Workspace4/1, MATLAB Function1/3(external_wrench), EQ generator/2(external_wrench), Scope5/1, BallBot Plant1/2(wrench_ext)  "external wrench"
  LQR Controller1/3(tau_r) -> Scope3/1
  Constant6/1 -> LQR Controller1/2(waypoints)
  LQR Controller1/1(tau) -> Scope9/1, To Workspace1/1
  PS-Simulink Converter1/1 -> Demux2/1, Scope4/1
  Demux2/2 -> Mux4/2
  Demux2/1 -> Mux4/1
  Mux4/1 -> Mux2/1
  LQR Controller1/5(tau_ff) -> Scope1/1
  EQ generator/1(theta_EQ) -> Hybrid Compensated LQR-PI Control/3(theta_EQ)
  EQ generator/2(tau_EQ) -> Hybrid Compensated LQR-PI Control/4(tau_EQ)
  Hybrid Compensated LQR-PI Control/1(tau) -> BallBot Plant1/1(tau), To Workspace7/1
  Clock1/1 -> Hybrid Compensated LQR-PI Control/5(sim_time)
  Clock2/1 -> MATLAB Function/3(simtime)
  Gain1/1 -> Demux3/1
  Demux3/1 -> Atan2/2
  MATLAB Function/1(phi_dot_c) -> Scope10/1, Hybrid Compensated LQR-PI Control/2(dot_phi_cmd), EQ generator/1(phi_dot_c), Gain1/1
  Atan2/1 -> MATLAB Function1/1(alpha_traj)
  [theta_z] -> MATLAB Function1/2(thetaz)
  MATLAB Function1/1(thetaz_des) -> Hybrid Compensated LQR-PI Control/6(thetaz_des), Scope7/1
  Gain2/1 -> Atan2/1
  Demux3/2 -> Gain2/1
  Constant1/1 -> MATLAB Function/2(waypoints)
  MATLAB Function/2(is_final_segment) -> Hybrid Compensated LQR-PI Control/7(is_final_segment)
  Clock/1 -> Time Scheduling/1
  1-D Lookup Table/1 -> [shoulder_pan_traj]
  1-D Lookup Table1/1 -> [shoulder_lift_traj]
  1-D Lookup Table2/1 -> [elbow_joint_traj]
  1-D Lookup Table3/1 -> [robotiq_traj]
  1-D Lookup Table4/1 -> [wrist_1_traj]
  1-D Lookup Table5/1 -> [wrist_2_traj]
  1-D Lookup Table6/1 -> [wrist_3_traj]
  [shoulder_pan_traj] -> Simulink-PS Converter2/1, Scope12/1
  [shoulder_lift_traj] -> Simulink-PS Converter3/1
  [wrist_1_traj] -> Simulink-PS Converter5/1
  [wrist_2_traj] -> Simulink-PS Converter6/1
  [wrist_3_traj] -> Simulink-PS Converter7/1
  Hybrid Compensated LQR-PI Control/2(is_ballbot_motion_finished) -> [is_ballbot_motion_finished], Display/1, Clock/1
  [elbow_joint_traj] -> Simulink-PS Converter4/1
  Time Scheduling/1 -> 1-D Lookup Table6/1, 1-D Lookup Table5/1, 1-D Lookup Table4/1, 1-D Lookup Table3/1, 1-D Lookup Table2/1, 1-D Lookup Table1/1, 1-D Lookup Table/1, [manip_time], Scope/1
  [T_desired] -> OP SPACE CONTROLLER/1(T_desired)
  OP SPACE CONTROLLER/2(error_pos) -> To Workspace10/1, Scope17/1
  BallBot Plant1/1(x) -> OP SPACE CONTROLLER/2(x_ballbot), Demux1/1, To Workspace/1, Hybrid Compensated LQR-PI Control/1(x), MATLAB Function/1(x)
  [q_manip] -> OP SPACE CONTROLLER/3(q_manip_actual)
  [manip_time] -> Smart LookUpTable/1(t_in)
  Smart LookUpTable/1(T_desired) -> [T_desired]
  Memory/1 -> Max/2
  Max/1 -> Display3/1, [manipulating], Memory/1
  [is_ballbot_motion_finished] -> Max/1
  [manipulating] -> OP SPACE CONTROLLER/Enable
  Hybrid Compensated LQR-PI Control/3(distance_to_goal) -> Scope13/1
  Mux3/1 -> MATLAB Function2/1(x)
  MATLAB Function2/1(h_base) -> Simulink-PS Converter9/1
  Demux1/2 -> Mux3/2, Simulink-PS Converter11/1
  Demux1/1 -> Mux3/1, Simulink-PS Converter10/1
  MATLAB Function/3(position_error) -> To Workspace11/1
  connections:
  robotiq_85_left_knuckle_joint/RConn1 -- robotiq_85_left_knuckle_link/LConn1
  robotiq_85_base_link/RConn3 -- robotiq_85_left_knuckle_joint/LConn1
  flange_tool0/RConn1 -- tool0/LConn1
  robotiq_85_base_joint/RConn1 -- robotiq_85_base_link/LConn1
  robotiq_85_base_link/RConn1 -- robotiq_85_right_knuckle_joint/LConn1
  robotiq_85_base_link/RConn2 -- robotiq_85_right_inner_knuckle_joint/LConn1
  robotiq_85_left_knuckle_joint/RConn2 -- PS Gain1/LConn1 -- PS Gain/LConn1 -- PS Gain2/LConn1
  robotiq_85_base_link/RConn4 -- robotiq_85_left_inner_knuckle_joint/LConn1
  robotiq_85_left_inner_knuckle_joint/RConn1 -- robotiq_85_left_inner_knuckle_link/LConn1
  PS Gain/RConn1 -- robotiq_85_right_inner_knuckle_joint/LConn2
  PS Gain1/RConn1 -- robotiq_85_right_knuckle_joint/LConn2
  robotiq_85_left_knuckle_link/RConn1 -- robotiq_85_left_finger_joint/LConn1
  Simulink-PS Converter13/RConn1 -- Gimbal Joint/LConn4
  base_joint/RConn1 -- base_link/LConn1
  robotiq_85_right_knuckle_joint/RConn1 -- robotiq_85_right_knuckle_link/LConn1
  robotiq_85_left_finger_joint/RConn1 -- robotiq_85_left_finger_link/LConn1
  wrist_1_link/RConn1 -- wrist_2_joint/LConn1
  robotiq_85_right_inner_knuckle_joint/RConn1 -- robotiq_85_right_inner_knuckle_link/LConn1
  PS Gain2/RConn1 -- robotiq_85_left_finger_tip_joint/LConn2
  robotiq_85_right_knuckle_link/RConn1 -- robotiq_85_right_finger_joint/LConn1
  robotiq_85_left_finger_link/RConn1 -- robotiq_85_left_finger_tip_joint/LConn1
  robotiq_85_right_finger_joint/RConn1 -- robotiq_85_right_finger_link/LConn1
  robotiq_85_left_finger_tip_joint/RConn1 -- robotiq_85_left_finger_tip_link/LConn1
  robotiq_85_right_finger_link/RConn1 -- robotiq_85_right_finger_tip_joint/LConn1
  robotiq_85_right_finger_tip_joint/RConn1 -- robotiq_85_right_finger_tip_link/LConn1
  base_link/RConn1 -- base_link_base_link_inertia/LConn1
  base_link/RConn2 -- base_link_base_fixed_joint/LConn1
  wrist_3_link/RConn1 -- wrist_3_link_ft_frame/LConn1
  base_link_base_link_inertia/RConn1 -- base_link_inertia/LConn1
  base_link_base_fixed_joint/RConn1 -- base/LConn1
  Simulink-PS Converter/RConn1 -- Cartesian Joint/LConn2
  base_link_inertia/RConn1 -- shoulder_pan_joint/LConn1
  shoulder_pan_joint/RConn1 -- shoulder_link/LConn2
  shoulder_link/RConn1 -- shoulder_lift_joint/LConn1
  Simulink-PS Converter8/RConn1 -- Cartesian Joint/LConn3
  shoulder_lift_joint/RConn1 -- upper_arm_link/LConn1
  upper_arm_link/RConn1 -- elbow_joint/LConn1
  elbow_joint/RConn1 -- forearm_link/LConn1
  wrist_2_link/RConn1 -- wrist_3_joint/LConn1
  forearm_link/RConn1 -- wrist_1_joint/LConn1
  wrist_1_joint/RConn1 -- wrist_1_link/LConn1
  wrist_2_joint/RConn1 -- wrist_2_link/LConn1
  wrist_3_joint/RConn1 -- wrist_3_link/LConn1
  wrist_3_link/RConn2 -- wrist_3_flange/LConn1
  wrist_3_link_ft_frame/RConn1 -- ft_frame/LConn1
  wrist_3_flange/RConn1 -- flange/LConn1
  Simulink-PS Converter10/RConn1 -- Gimbal Joint/LConn2
  world/RConn1 -- ground_plane_joint/LConn1
  world/RConn2 -- Cartesian Joint/LConn1
  Simulink-PS Converter9/RConn1 -- Cartesian Joint/LConn4
  World/RConn1 -- MechanismConfiguration/RConn1 -- Solver Configuration/RConn1 -- world/LConn1
  ground_plane_joint/RConn1 -- ground_plane/LConn1
  Simulink-PS Converter11/RConn1 -- Gimbal Joint/LConn3
  Cartesian Joint/RConn1 -- Gimbal Joint/LConn1
  flange/RConn2 -- flange_tool0/LConn1
  flange/RConn1 -- robotiq_85_base_joint/LConn1
  ground_plane/RConn5 -- wrist_2_link/LConn2
  ground_plane/RConn1 -- shoulder_link/LConn1
  ground_plane/RConn2 -- upper_arm_link/LConn2
  ground_plane/RConn3 -- forearm_link/LConn2
  ground_plane/RConn4 -- wrist_1_link/LConn2
  ground_plane/RConn6 -- wrist_3_link/LConn2
  Gimbal Joint/RConn1 -- base_joint/LConn1
  PS-Simulink Converter1/LConn1 -- Cartesian Joint/RConn2
  PS-Simulink Converter2/LConn1 -- Gimbal Joint/RConn2
  PS-Simulink Converter/LConn1 -- shoulder_pan_joint/RConn2
  shoulder_pan_joint/LConn2 -- Simulink-PS Converter2/RConn1
  shoulder_lift_joint/RConn2 -- PS-Simulink Converter3/LConn1
  shoulder_lift_joint/LConn2 -- Simulink-PS Converter3/RConn1
  PS-Simulink Converter4/LConn1 -- elbow_joint/RConn2
  wrist_1_joint/RConn2 -- PS-Simulink Converter5/LConn1
  wrist_2_joint/RConn2 -- PS-Simulink Converter6/LConn1
  wrist_3_joint/RConn2 -- PS-Simulink Converter7/LConn1
  elbow_joint/LConn2 -- Simulink-PS Converter4/RConn1
  Simulink-PS Converter1/RConn1 -- robotiq_85_right_finger_tip_joint/LConn2 -- robotiq_85_left_inner_knuckle_joint/LConn2 -- robotiq_85_left_knuckle_joint/LConn2
  wrist_1_joint/LConn2 -- Simulink-PS Converter5/RConn1
  wrist_2_joint/LConn2 -- Simulink-PS Converter6/RConn1
  wrist_3_joint/LConn2 -- Simulink-PS Converter7/RConn1
  shoulder_pan_joint/RConn3 -- PS-Simulink Converter8/LConn1
  shoulder_lift_joint/RConn3 -- PS-Simulink Converter9/LConn1
  elbow_joint/RConn3 -- PS-Simulink Converter10/LConn1
  wrist_1_joint/RConn3 -- PS-Simulink Converter11/LConn1
  wrist_2_joint/RConn3 -- PS-Simulink Converter12/LConn1
  wrist_3_joint/RConn3 -- PS-Simulink Converter13/LConn1

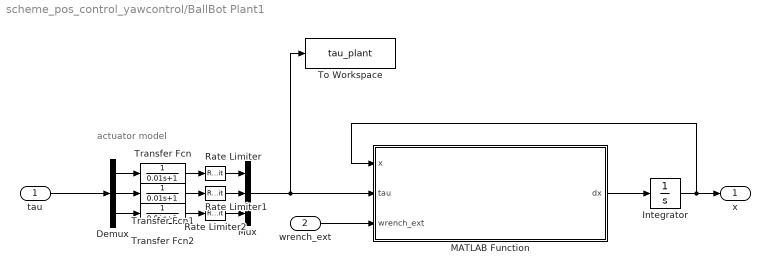
== system scheme_pos_control_yawcontrol/BallBot Plant1 ==
  note: actuator model
  tau : Inport
  wrench_ext : Inport  Port=2
  Demux : Demux  Outputs=3
  Integrator : Integrator  InitialCondition=x0(1:10)
  MATLAB Function : MATLAB Function  TreatAsAtomicUnit=on
  Mux : Mux  Inputs=3
  Rate Limiter : RateLimiter  RisingSlewLimit=100  FallingSlewLimit=-100  SampleTimeMode=inherited
  Rate Limiter1 : RateLimiter  RisingSlewLimit=100  FallingSlewLimit=-100  SampleTimeMode=inherited
  Rate Limiter2 : RateLimiter  RisingSlewLimit=100  FallingSlewLimit=-100  SampleTimeMode=inherited
  To Workspace : ToWorkspace  VariableName=tau_plant  SaveFormat=Timeseries  SampleTime=-1
  Transfer Fcn : TransferFcn  Denominator=[0.01 1]
  Transfer Fcn1 : TransferFcn  Denominator=[0.01 1]
  Transfer Fcn2 : TransferFcn  Denominator=[0.01 1]
  x : Outport
  wires:
  MATLAB Function/1(dx) -> Integrator/1
  Integrator/1 -> MATLAB Function/1(x), x/1
  wrench_ext/1 -> MATLAB Function/3(wrench_ext)
  tau/1 -> Demux/1
  Demux/1 -> Transfer Fcn/1
  Demux/2 -> Transfer Fcn1/1
  Demux/3 -> Transfer Fcn2/1
  Transfer Fcn/1 -> Rate Limiter/1
  Rate Limiter/1 -> Mux/1
  Transfer Fcn1/1 -> Rate Limiter1/1
  Rate Limiter1/1 -> Mux/2
  Transfer Fcn2/1 -> Rate Limiter2/1
  Rate Limiter2/1 -> Mux/3
  Mux/1 -> To Workspace/1, MATLAB Function/2(tau)

== system scheme_pos_control_yawcontrol/OP SPACE CONTROLLER ==
  T_desired : Inport
  x_ballbot : Inport  Port=2
  q_manip_actual : Inport  Port=3
  Enable : EnablePort
  MATLAB Function3 : MATLAB Function  TreatAsAtomicUnit=on
  q_dot_command : Outport
  error_pos : Outport  Port=2
  wires:
  T_desired/1 -> MATLAB Function3/1(T_desired)
  q_manip_actual/1 -> MATLAB Function3/3(q_manip_actual)
  MATLAB Function3/1(q_dot_command) -> q_dot_command/1
  x_ballbot/1 -> MATLAB Function3/2(x_ballbot)
  MATLAB Function3/2(error_pos) -> error_pos/1
